simulink model "test_kalman_filter"  (R2018a)
settings: Solver=FixedStepAuto  StartTime=0.0  StopTime=200  RelTol=1e-3
values from neighbouring files (symbols this model uses):
  dt = 1/100    (= 0.01)    [parameters.m]
  P0 = [1e-06 0 0;0 1e-06 0;0 0 1e-06]    [parameters.m]
  Q = diag([a*pqr_dot_covar(1)*a, a*pqr_dot_covar(2)*a, a*pqr_dot_covar(3)*a])    [parameters.m]
  R = diag([0.1, 0.1, 0.1])*9.81    [parameters.m]
  x0 = [0;0;0]    [parameters.m]
undefined symbols (not defined in the file or in its folder): lpfDtDen, lpfDtNum
libraries: myLib x3, simulink_extras x3, sharedtransform x1
settings Model: Creator=Test  LastModifiedBy=Test

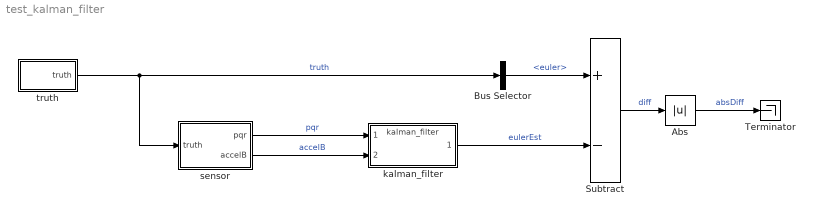
== system test_kalman_filter ==
  Abs : Abs
  Bus Selector : BusSelector  OutputSignals=euler
  Subtract : Sum  Inputs=+-
  Terminator : Terminator
  kalman_filter : ModelReference  ModelNameDialog=kalman_filter  ParameterArgumentNames=P0,Q,R,dt,x0  ParameterArgumentValues=P0,Q,R,dt,x0  UsingDefaultArgumentValue=0,0,0,0,0  SimulationMode=Normal  ModelReferenceVersion=1.255
  sensor : Subsystem
  truth : Subsystem
  wires:
  Abs/1 -> Terminator/1  "absDiff"
  kalman_filter/1 -> Subtract/2  "eulerEst"
  truth/1(truth) -> Bus Selector/1, sensor/1(truth)  "truth"
  Bus Selector/1 -> Subtract/1  "<euler>"
  sensor/2(accelB) -> kalman_filter/2  "accelB"
  sensor/1(pqr) -> kalman_filter/1  "pqr"
  Subtract/1 -> Abs/1  "diff"

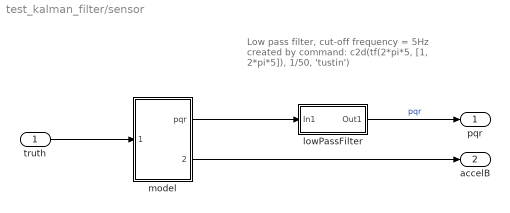
== system test_kalman_filter/sensor ==
  note: Low pass filter, cut-off frequency = 5Hz
      |
      | created by command:
      | c2d(tf(2*pi*5, [1, 2*pi*5]), 1/50, 'tustin')
  truth : Inport
  lowPassFilter : Subsystem  mask{Numerator=lpfDtNum{1}, Denominator=lpfDtDen{1}, SampleTime=-1}
      mask prompts: Numerator "Simulink:blkprm_prompts:FilterTFNumerator"; Denominator "Simulink:blkprm_prompts:FilterTFDenominator"; SampleTime "Simulink:blkprm_prompts:AllBlksSampleTime"
      mask TypeOptions Numerator:
      | Discrete
      | Transfer Fcn/Numerator | Discrete
      | Transfer Fcn1/Numerator | Discrete
      | Transfer Fcn2/Numerator
      mask TypeOptions Denominator:
      | Discrete
      | Transfer Fcn/Denominator | Discrete
      | Transfer Fcn1/Denominator | Discrete
      | Transfer Fcn2/Denominator
      mask TypeOptions SampleTime:
      | Discrete
      | Transfer Fcn/SampleTime | Discrete
      | Transfer Fcn1/SampleTime | Discrete
      | Transfer Fcn2/SampleTime
      mask DialogControl Numerator Prompt: Numerator coefficients:
      mask DialogControl Denominator Prompt: Denominator coefficients:
      mask DialogControl SampleTime Prompt: Sample time (-1 for inherited):
  model : Subsystem  mask{SampleTime=1/100}
      mask prompts: SampleTime "Simulink:blkprm_prompts:AllSrcBlksSampleTime"
      mask TypeOptions SampleTime:
      | Random
      | Number/SampleTime | Random
      | Number1/SampleTime | Rate Transition/OutPortSampleTime | Rate Transition1/OutPortSampleTime
      mask DialogControl SampleTime Prompt: Sample time:
  pqr : Outport
  accelB : Outport  Port=2
  wires:
  lowPassFilter/1(Out1) -> pqr/1  "pqr"
  truth/1 -> model/1(truth)
  model/1(pqr) -> lowPassFilter/1(In1)
  model/2(accelB) -> accelB/1

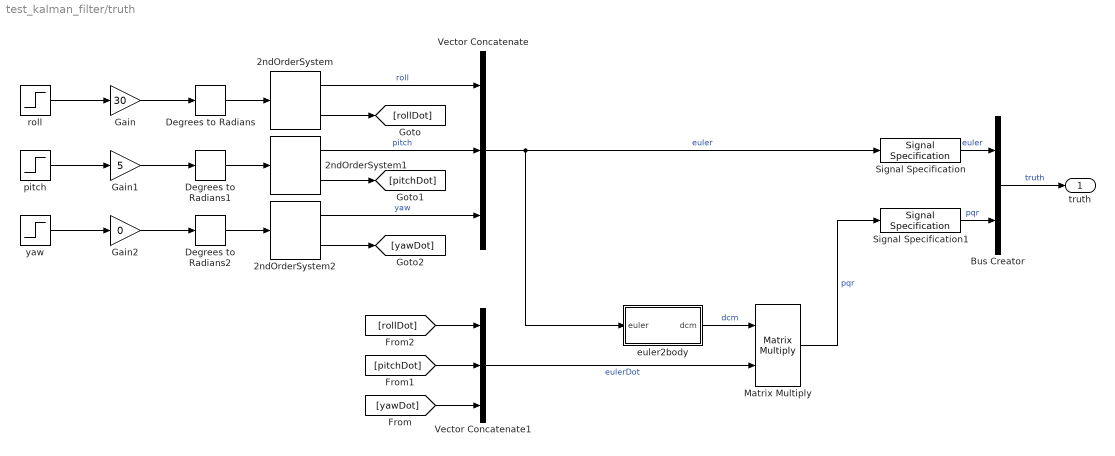
== system test_kalman_filter/truth ==
  2ndOrderSystem : myLib/2ndOrderSystem  wn=1  zeta=0.707  p0=0  v0=0
  2ndOrderSystem1 : myLib/2ndOrderSystem  wn=1  zeta=0.707  p0=0  v0=0
  2ndOrderSystem2 : myLib/2ndOrderSystem  wn=1  zeta=0.707  p0=0  v0=0
  Bus Creator : BusCreator  Inputs=2
  Degrees to Radians : simulink_extras/Transformations/Degrees to Radians
  Degrees to Radians1 : simulink_extras/Transformations/Degrees to Radians
  Degrees to Radians2 : simulink_extras/Transformations/Degrees to Radians
  Gain : Gain  Gain=30
  Gain1 : Gain  Gain=5
  Gain2 : Gain  Gain=0
  Matrix Multiply : Product  Multiplication=Matrix(*)
  Signal Specification : SignalSpecification  Unit=rad  Dimensions=3
  Signal Specification1 : SignalSpecification  Unit=rad/s  Dimensions=3
  Vector Concatenate : Concatenate  NumInputs=3
  Vector Concatenate1 : Concatenate  NumInputs=3
  euler2body : MATLAB Function  TreatAsAtomicUnit=on
  pitch : Step  SampleTime=0
  roll : Step  SampleTime=0
  yaw : Step  SampleTime=0
  truth : Outport
  wires:
  Degrees to Radians/1 -> 2ndOrderSystem/1
  Degrees to Radians1/1 -> 2ndOrderSystem1/1
  2ndOrderSystem2/1 -> Vector Concatenate/3  "yaw"
  2ndOrderSystem1/1 -> Vector Concatenate/2  "pitch"
  Degrees to Radians2/1 -> 2ndOrderSystem2/1
  roll/1 -> Gain/1
  yaw/1 -> Gain2/1
  pitch/1 -> Gain1/1
  2ndOrderSystem/1 -> Vector Concatenate/1  "roll"
  Vector Concatenate/1 -> euler2body/1(euler), Signal Specification/1  "euler"
  Bus Creator/1 -> truth/1  "truth"
  2ndOrderSystem/2 -> [rollDot]
  2ndOrderSystem1/2 -> [pitchDot]
  2ndOrderSystem2/2 -> [yawDot]
  [pitchDot] -> Vector Concatenate1/2
  [rollDot] -> Vector Concatenate1/1
  [yawDot] -> Vector Concatenate1/3
  Vector Concatenate1/1 -> Matrix Multiply/2  "eulerDot"
  Matrix Multiply/1 -> Signal Specification1/1  "pqr"
  euler2body/1(dcm) -> Matrix Multiply/1  "dcm"
  Signal Specification/1 -> Bus Creator/1  "euler"
  Signal Specification1/1 -> Bus Creator/2  "pqr"
  Gain/1 -> Degrees to Radians/1
  Gain1/1 -> Degrees to Radians1/1
  Gain2/1 -> Degrees to Radians2/1

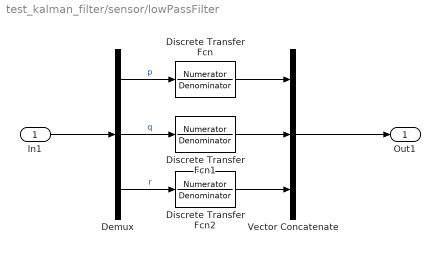
== system test_kalman_filter/sensor/lowPassFilter ==
  In1 : Inport
  Demux : Demux  Outputs=3
  Discrete Transfer Fcn : DiscreteTransferFcn  Numerator=Numerator  Denominator=Denominator  SampleTime=SampleTime
  Discrete Transfer Fcn1 : DiscreteTransferFcn  Numerator=Numerator  Denominator=Denominator  SampleTime=SampleTime
  Discrete Transfer Fcn2 : DiscreteTransferFcn  Numerator=Numerator  Denominator=Denominator  SampleTime=SampleTime
  Vector Concatenate : Concatenate  NumInputs=3
  Out1 : Outport
  wires:
  Vector Concatenate/1 -> Out1/1
  Discrete Transfer Fcn1/1 -> Vector Concatenate/2
  Discrete Transfer Fcn2/1 -> Vector Concatenate/3
  Discrete Transfer Fcn/1 -> Vector Concatenate/1
  In1/1 -> Demux/1
  Demux/1 -> Discrete Transfer Fcn/1  "p"
  Demux/3 -> Discrete Transfer Fcn2/1  "r"
  Demux/2 -> Discrete Transfer Fcn1/1  "q"

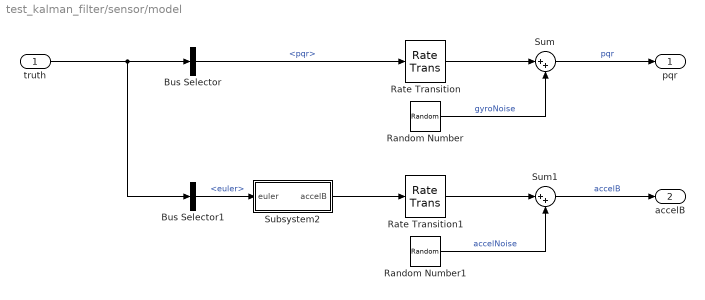
== system test_kalman_filter/sensor/model ==
  truth : Inport
  Bus Selector : BusSelector  OutputSignals=pqr
  Bus Selector1 : BusSelector  OutputSignals=euler
  Random Number : RandomNumber  Variance=[deg2rad(1)^2, deg2rad(1)^2, deg2rad(1)^2]  Seed=[23341, 23342, 23343]  SampleTime=SampleTime
  Random Number1 : RandomNumber  Variance=9.81*[0.1^2, 0.1^2, 0.1^2]  Seed=[23351, 23352, 23353]  SampleTime=SampleTime
  Rate Transition : RateTransition  OutPortSampleTime=SampleTime
  Rate Transition1 : RateTransition  OutPortSampleTime=SampleTime
  Subsystem2 : Subsystem
  Sum : Sum  Inputs=|++
  Sum1 : Sum  Inputs=|++
  pqr : Outport
  accelB : Outport  Port=2
  wires:
  truth/1 -> Bus Selector1/1, Bus Selector/1
  Random Number/1 -> Sum/2  "gyroNoise"
  Random Number1/1 -> Sum1/2  "accelNoise"
  Subsystem2/1(accelB) -> Rate Transition1/1
  Bus Selector/1 -> Rate Transition/1  "<pqr>"
  Bus Selector1/1 -> Subsystem2/1(euler)  "<euler>"
  Sum1/1 -> accelB/1  "accelB"
  Sum/1 -> pqr/1  "pqr"
  Rate Transition/1 -> Sum/1
  Rate Transition1/1 -> Sum1/1

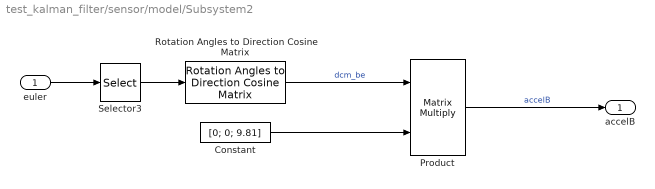
== system test_kalman_filter/sensor/model/Subsystem2 ==
  euler : Inport
  Constant : Constant  Value=[0; 0; 9.81]
  Product : Product  Multiplication=Matrix(*)
  Rotation Angles to Direction Cosine Matrix : sharedtransform/Rotation Angles to Direction Cosine Matrix  rotationOrder=ZYX  aMode=aMode
      settings: SourceProductBaseCode=AE
  Selector3 : Selector  InputPortWidth=3  IndexOptions=Index vector (dialog)  Indices=[3 2 1]  OutputSizes=1
  accelB : Outport
  wires:
  euler/1 -> Selector3/1
  Rotation Angles to Direction Cosine Matrix/1 -> Product/1  "dcm_be"
  Product/1 -> accelB/1  "accelB"
  Constant/1 -> Product/2
  Selector3/1 -> Rotation Angles to Direction Cosine Matrix/1

== matlab function test_kalman_filter/truth/euler2body ==
  data: dcm output; euler input
function dcm = fcn(euler)

phi = euler(1);
theta = euler(2);

% body to euler
% dcm = [
%     1 sin(phi)*tan(theta) cos(phi)*tan(theta);
%     0 cos(phi) -sin(phi);
%     0 sin(phi)*sec(theta) cos(phi)*sec(theta)];

% euler to body
dcm = [
    1 0 -sin(theta);
    0 cos(phi) sin(phi)*cos(theta);
    0 -sin(phi) cos(phi)*cos(theta)];

end
